simulink model "car_pendulum_model"  (R2020b)
settings: Solver=VariableStepAuto  StartTime=0.0  StopTime=10.0  RelTol=1e-3
settings Model: Creator=petir  LastModifiedBy=petir

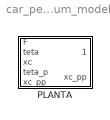
== system car_pendulum_model ==
  PLANTA : MATLAB Function  TreatAsAtomicUnit=on

== matlab function car_pendulum_model/PLANTA ==
  data: F input; teta_pp output; teta input; xc input; teta_p input; xc_pp input; xc_pp output
function [teta_pp, xc_pp] = fcn(F, teta, xc, teta_p, xc_pp)
m = 1;
M = 2;
l = 0.5;
L = 1;
g = 9.81;

det = ((M + m)*m*l^2 - (m*l*cos(teta))^2);

xc_pp = (m*l^2 * (F + m*l*sin(teta) * teta_p^2)... 
            - m*l*cos(teta) * (m*g*l*sin(teta))) / det;
teta_pp = (-m*l*cos(teta) * (F + m*l*sin(teta) * teta_p^2)...
            + (M + m)*(m*g*l*sin(teta))) / det;
